simulink model "softarm_actuator_acceleration_block"  (R2025a)
settings: Solver=ode15s  StartTime=0.0  StopTime=1  RelTol=1e-3
PreLoadFcn:
  | softarm_model_dir=fileparts(get_param(bdroot,'FileName'));softarm_root=fileparts(fileparts(softarm_model_dir));addpath(fullfile(softarm_root,'matlab'));addpath(fullfile(softarm_root,'matlab','simulink'));
InitFcn:
  | softarm_model_dir=fileparts(get_param(bdroot,'FileName'));softarm_root=fileparts(fileparts(softarm_model_dir));addpath(fullfile(softarm_root,'matlab'));addpath(fullfile(softarm_root,'matlab','simulink'));if evalin('base','exist(''softarm_bundle'',''var'')'),softarm_selected_bundle=evalin('base','softarm_bundle');else,softarm_selected_bundle=fullfile(softarm_root,'examples','generated','extensible_euler_bernoulli_pcs_three_tendon_n2');end;softarm_loaded=softarm.initModel(string(softarm_selected_bundle));assert(~isempty(softarm_loaded.actuation),'softarm:MissingActuation','Selected bundle has no actuator mapping.');assert(isfield(softarm_loaded.actuation,'acceleration'),'softarm:MissingAcceleration','Selected bundle has no strict acceleration mapping.');
undefined symbols (not defined in the file): softarm_p
settings Model: Creator=rlwan  LastModifiedBy=rlwan

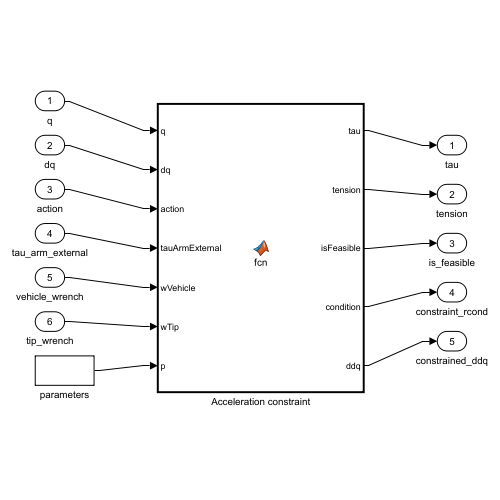
[thumbnail: Simulink's stored preview of the top-level diagram]
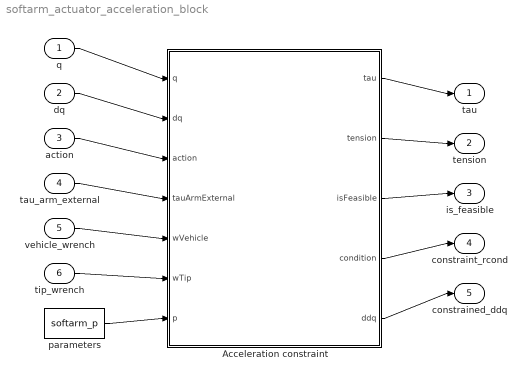
== system softarm_actuator_acceleration_block ==
  q : Inport  PortDimensions=softarm_nq
  dq : Inport  Port=2  PortDimensions=softarm_nq
  action : Inport  Port=3  PortDimensions=softarm_nu
  tau_arm_external : Inport  Port=4  PortDimensions=softarm_narm
  vehicle_wrench : Inport  Port=5  PortDimensions=6
  tip_wrench : Inport  Port=6  PortDimensions=6
  Acceleration constraint : MATLAB Function  TreatAsAtomicUnit=on
  parameters : Constant  Value=softarm_p
  tau : Outport
  tension : Outport  Port=2
  is_feasible : Outport  Port=3
  constraint_rcond : Outport  Port=4
  constrained_ddq : Outport  Port=5
  wires:
  q/1 -> Acceleration constraint/1(q)
  dq/1 -> Acceleration constraint/2(dq)
  action/1 -> Acceleration constraint/3(action)
  tau_arm_external/1 -> Acceleration constraint/4(tauArmExternal)
  vehicle_wrench/1 -> Acceleration constraint/5(wVehicle)
  tip_wrench/1 -> Acceleration constraint/6(wTip)
  parameters/1 -> Acceleration constraint/7(p)
  Acceleration constraint/1(tau) -> tau/1
  Acceleration constraint/2(tension) -> tension/1
  Acceleration constraint/3(isFeasible) -> is_feasible/1
  Acceleration constraint/4(condition) -> constraint_rcond/1
  Acceleration constraint/5(ddq) -> constrained_ddq/1

== matlab function softarm_actuator_acceleration_block/Acceleration constraint ==
  data: q input; tau output; dq input; action input; tauArmExternal input; wVehicle input; wTip input; p input; tension output; isFeasible output; condition output; ddq output
function [tau,tension,isFeasible,condition,ddq] = fcn(q,dq,action,tauArmExternal,wVehicle,wTip,p)
%#codegen
[ddq,tension,isFeasible,condition]=softarm_actuator_acceleration(q,dq,action,tauArmExternal,wVehicle,wTip,p);
Ja=softarm_actuator_jacobian(q,p);
tau=tauArmExternal-Ja.'*tension;
end
